simulink model "darko_control_lineaire_lqi"  (R2021b)
settings: Solver=VariableStepAuto  StartTime=0.0  StopTime=30  RelTol=1e-3
values from neighbouring files (symbols this model uses):
  drone = generateDarko()    [main_linearisation.m]
  initial_state = [p_initial; v_initial; q_initial; omega_initial]    [main_linearisation.m]
  K_complet_i = [Ki(:,1:6), zeros(4,1), Ki(:,7:15)]    [main_linearisation.m]
  S_complet_i = [Si(1:6,1:6), zeros(6,1), Si(1:6,7:15); zeros(1,16); Si(7:15,1:6), zeros(9,1), Si(7:15,7:15)]    [main_linearisation.m]
  u_eq = drone.G*drone.MASS/(2*drone.Fb(1,1)) * [1;1;0;0]    [main_linearisation.m]
  x_eq = [[0; 0; 0]; [0; 0; 0]; eul2quat([yaw, pitch, roll])'; [0; 0; 0]]    [main_linearisation.m]
libraries: simulink_extras x11, aerolibanim x1, sharedtransform x1
settings Model: Creator=florian  LastModifiedBy=florian
settings SolverCC: AlgebraicLoopSolver=TrustRegion
settings DebuggingCC: SFMachineParentedDataDiag=warning

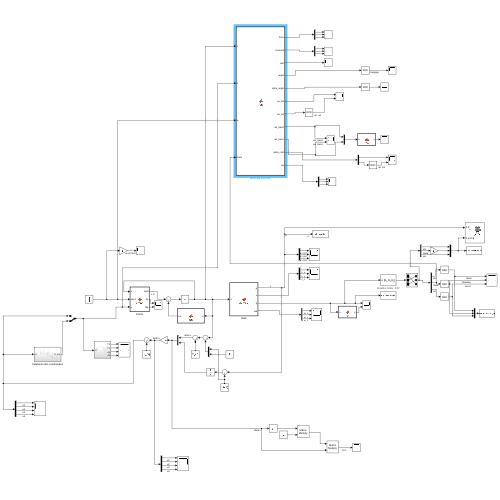
[thumbnail: Simulink's stored preview of the top-level diagram]
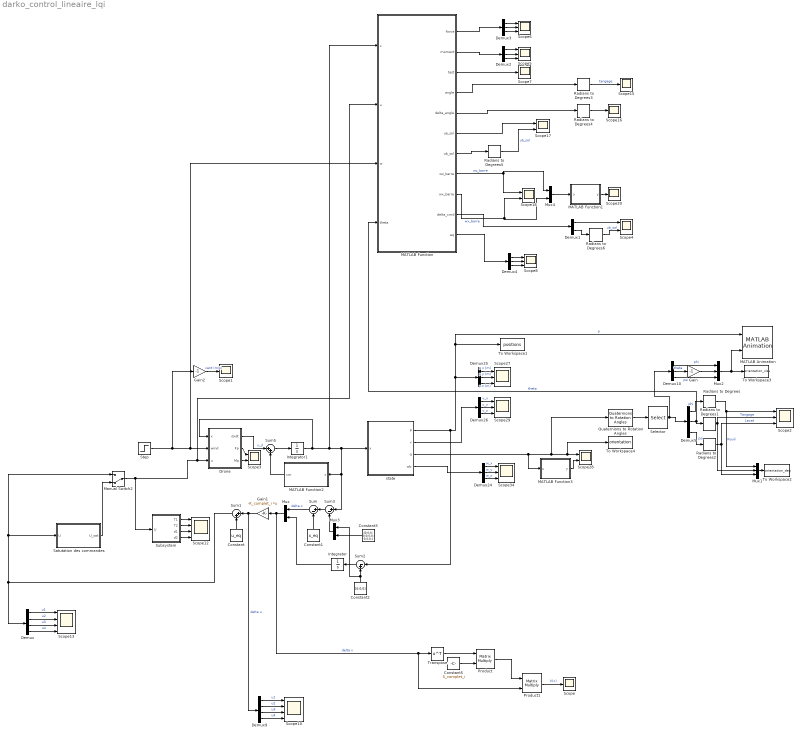
== system darko_control_lineaire_lqi ==
  Constant : Constant  Value=u_eq
  Constant1 : Constant  Value=x_eq
  Constant2 : Constant  Value=[0;0;0]
  Constant3 : Constant  Value=[0;0;0; 0;0;0;0; 0;0;0;]
  Constant5 : Constant  Value=S_complet_i
  Demux : Demux
  Demux1 : Demux  Outputs=2
  Demux{2..5,10,24..26} (8 alike) : Demux  Outputs=3
  Demux9 : Demux
  Drone : MATLAB Function  TreatAsAtomicUnit=on
  Gain : Gain  Gain=-1
  Gain1 : Gain  Gain=-K_complet_i  Multiplication=Matrix(K*u) (u vector)
  Gain2 : Gain  Gain=-1
  Integrator : Integrator  InitialCondition=[0;0;0]
  Integrator1 : Integrator  InitialCondition=initial_state
  MATLAB Animation : aerolibanim/MATLAB Animation  Tag=Matlab Animation 6 DOF  Vehicles=1  Geometries='astredwedge.mat'  BoundingBoxCoordinates=[-50,50,-50,50,-50,50]  CameraOffset=[0,-50,0]  CameraViewAngle=10  SampleTime=0.08  FigurePosition=[635,-23,492,413]
      settings: SourceProductBaseCode=AE
  MATLAB Function : MATLAB Function  TreatAsAtomicUnit=on
  MATLAB Function1 : MATLAB Function  TreatAsAtomicUnit=on
  MATLAB Function2 : MATLAB Function  TreatAsAtomicUnit=on
  MATLAB Function3 : MATLAB Function  TreatAsAtomicUnit=on
  Manual Switch2 : ManualSwitch  CurrentSetting=0
  Mux : Mux  Inputs=2
  Mux1 : Mux  Inputs=3
  Mux2 : Mux  Inputs=3
  Mux3 : Mux  Inputs=2
  Mux4 : Mux  Inputs=2
  Product : Product  Multiplication=Matrix(*)
  Product1 : Product  Multiplication=Matrix(*)
  Quaternions to Rotation Angles : sharedtransform/Quaternions to Rotation Angles  rotationOrder=ZXY  aMode=aMode
      settings: SourceProductBaseCode=AE,PW,DR,MT,UV,VE
  Radians to Degrees{,1..6} (7 alike) : simulink_extras/Transformations/Radians to Degrees
  Satutation des commandes : Subsystem
  Scope{,1,7,15..16,20} (6 alike) : Scope
  Scope10 : Scope  NumInputPorts=4
  Scope12 : Scope  NumInputPorts=4
  Scope13 : Scope  NumInputPorts=4
  Scope{3..4,17..18,28} (5 alike) : Scope  NumInputPorts=2
  Scope{2,5..6,8,27,29,34} (7 alike) : Scope  NumInputPorts=3
  Selector : Selector  InputPortWidth=3  IndexOptions=Index vector (dialog)  Indices=[2 3 1]  OutputSizes=1
  Step : Step  Time=10  Before=[0;0;0]  After=[-1;0;-1]  SampleTime=0
  Subsystem : Subsystem
  Sum : Sum  Inputs=|+-
  Sum1 : Sum  Inputs=|++
  Sum2 : Sum  Inputs=|-+
  Sum3 : Sum  Inputs=|+-
  Sum5 : Sum  Inputs=|++
  To Workspace1 : ToWorkspace  VariableName=positions  SampleTime=-1
  To Workspace2 : ToWorkspace  VariableName=orientation_deg  SampleTime=-1
  To Workspace3 : ToWorkspace  VariableName=orientation_visu  SampleTime=-1
  To Workspace4 : ToWorkspace  VariableName=orientation  SampleTime=-1
  Transpose : Math  Operator=transpose  SaturateOnIntegerOverflow=on
  state : MATLAB Function  TreatAsAtomicUnit=on
  wires:
  Sum5/1 -> Integrator1/1
  MATLAB Function2/1(cor) -> Sum5/2
  Drone/1(dxdt) -> Sum5/1  "x_d"
  Integrator1/1 -> Drone/1(x), MATLAB Function/1(x), state/1(x), Sum3/1, MATLAB Function2/1(x)
  Demux25/3 -> Scope27/3  "p z (m)"
  Demux26/2 -> Scope29/2  "v_y"
  Demux24/1 -> Scope34/1  "w_x"
  MATLAB Function3/1(y) -> Scope28/2
  Demux25/1 -> Scope27/1  "p x (m)"
  state/4(wb) -> Demux24/1
  Demux24/2 -> Scope34/2  "w_y"
  Demux24/3 -> Scope34/3  "w_z"
  state/2(v) -> Demux26/1
  Demux25/2 -> Scope27/2  "p y (m)"
  Demux26/3 -> Scope29/3  "v_z"
  Demux26/1 -> Scope29/1  "v_x"
  Constant/1 -> Sum1/2
  Constant1/1 -> Sum/2
  Demux9/3 -> Scope10/3  "u3"
  Demux9/4 -> Scope10/4  "u4"
  Demux9/1 -> Scope10/1  "u1"
  Demux9/2 -> Scope10/2  "u2"
  Step/1 -> Gain2/1, MATLAB Function/3(w), Drone/2(wind)
  Integrator/1 -> Mux/2
  Sum/1 -> Mux/1  "delta x"
  Demux5/2 -> Radians to Degrees1/1, MATLAB Function/4(theta)  "theta"
  Quaternions to Rotation Angles/1 -> Selector/1
  Demux5/1 -> Radians to Degrees/1  "phi"
  Demux5/3 -> Radians to Degrees2/1  "psi"
  Demux/3 -> Scope13/3  "u3"
  Sum1/1 -> Satutation des commandes/1(U), Manual Switch2/1, Demux/1
  Demux/2 -> Scope13/2  "u2"
  Demux/1 -> Scope13/1  "u1"
  Demux/4 -> Scope13/4  "u4"
  Product1/1 -> Scope/1  "V(x)"
  Gain1/1 -> Demux9/1, Sum1/1  "delta u"
  Product/1 -> Product1/1
  Transpose/1 -> Product/1
  Constant5/1 -> Product/2
  Mux/1 -> Product1/2, Transpose/1, Gain1/1  "delta x"
  Mux1/1 -> To Workspace2/1
  state/3(q) -> Scope28/1, To Workspace4/1, Quaternions to Rotation Angles/1, MATLAB Function3/1(u)
  Satutation des commandes/1(U_sat) -> Manual Switch2/2
  Demux10/2 -> Gain/1  "theta"
  Selector/1 -> Demux10/1, Demux5/1
  Gain/1 -> Mux2/2
  Demux10/1 -> Mux2/1  "phi"
  Demux10/3 -> Mux2/3  "psi"
  state/1(p) -> Sum2/1, Demux25/1, MATLAB Animation/1, To Workspace1/1  "p"
  Mux2/1 -> To Workspace3/1, MATLAB Animation/2
  Gain2/1 -> Scope1/1  "vent (m/s)"
  Radians to Degrees1/1 -> Scope2/2, Mux1/2  "Tangage"
  Radians to Degrees/1 -> Scope2/1, Mux1/1  "Rouli"
  Radians to Degrees2/1 -> Scope2/3, Mux1/3  "Lacet"
  Sum2/1 -> Integrator/1
  Constant2/1 -> Mux3/1, Sum2/2
  Sum3/1 -> Sum/1
  Mux3/1 -> Sum3/2
  Constant3/1 -> Mux3/2
  Drone/2(Fp) -> Scope3/1
  Drone/3(Mp) -> Scope3/2
  Manual Switch2/1 -> Subsystem/1(U), MATLAB Function/2(u), Drone/3(u)
  Subsystem/3(d1) -> Scope12/3
  Subsystem/4(d2) -> Scope12/4
  Subsystem/2(T2) -> Scope12/2
  Subsystem/1(T1) -> Scope12/1
  Mux4/1 -> MATLAB Function1/1(u)
  MATLAB Function/7(ub_sol) -> Radians to Degrees5/1
  MATLAB Function/5(delta_angle) -> Radians to Degrees4/1
  Radians to Degrees3/1 -> Scope15/1  "tangage"
  MATLAB Function1/1(y) -> Scope20/1
  MATLAB Function/4(angle) -> Radians to Degrees3/1
  Radians to Degrees4/1 -> Scope16/1
  Radians to Degrees5/1 -> Scope17/2  "ub_sol"
  MATLAB Function/9(wx_barre) -> Scope18/2, Mux4/2  "wx_barre"
  MATLAB Function/8(wz_barre) -> Scope18/1, Mux4/1  "wz_barre"
  MATLAB Function/6(ua_sol) -> Scope17/1
  MATLAB Function/10(delta_cmd) -> Demux1/1
  Demux1/1 -> Scope4/1
  Demux2/1 -> Scope5/1
  Demux2/2 -> Scope5/2
  Demux2/3 -> Scope5/3
  MATLAB Function/2(moment) -> Demux2/1
  Demux3/1 -> Scope6/1
  Demux3/2 -> Scope6/2
  Demux3/3 -> Scope6/3
  MATLAB Function/1(force) -> Demux3/1
  MATLAB Function/3(test) -> Scope7/1
  Radians to Degrees6/1 -> Scope4/2  "ub_sol"
  Demux1/2 -> Radians to Degrees6/1
  Demux4/1 -> Scope8/1
  Demux4/2 -> Scope8/2
  Demux4/3 -> Scope8/3
  MATLAB Function/11(eq) -> Demux4/1

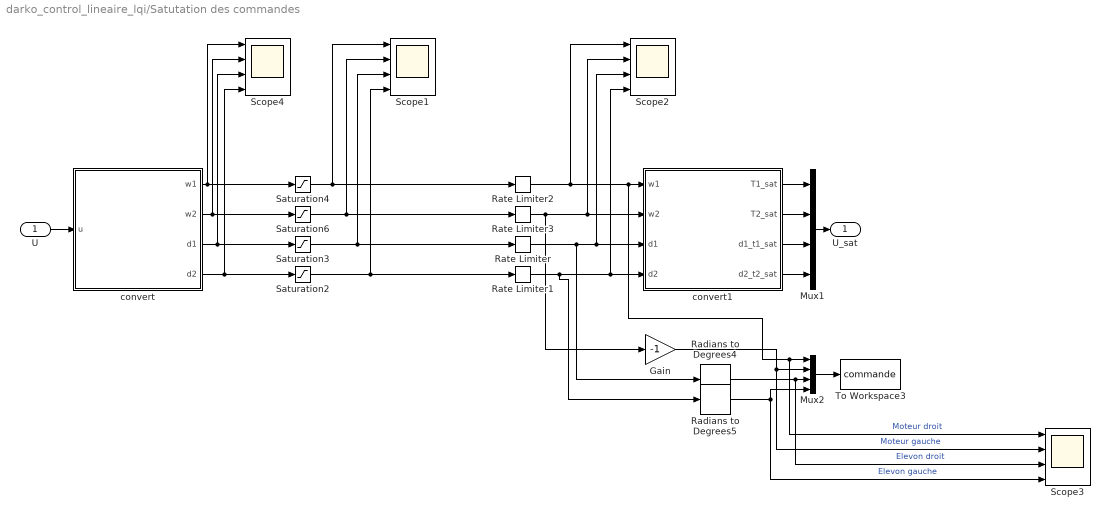
== system darko_control_lineaire_lqi/Satutation des commandes ==
  U : Inport
  Gain : Gain  Gain=-1
  Mux1 : Mux
  Mux2 : Mux
  Radians to Degrees4 : simulink_extras/Transformations/Radians to Degrees
  Radians to Degrees5 : simulink_extras/Transformations/Radians to Degrees
  Rate Limiter : RateLimiter  RisingSlewLimit=drone.ELEVON_RATE_CHANGE  FallingSlewLimit=-drone.ELEVON_RATE_CHANGE  SampleTimeMode=inherited
  Rate Limiter1 : RateLimiter  RisingSlewLimit=drone.ELEVON_RATE_CHANGE  FallingSlewLimit=-drone.ELEVON_RATE_CHANGE  SampleTimeMode=inherited
  Rate Limiter2 : RateLimiter  RisingSlewLimit=drone.MOTOR_RATE_CHANGE  FallingSlewLimit=-drone.MOTOR_RATE_CHANGE  SampleTimeMode=inherited
  Rate Limiter3 : RateLimiter  RisingSlewLimit=drone.MOTOR_RATE_CHANGE  FallingSlewLimit=-drone.MOTOR_RATE_CHANGE  SampleTimeMode=inherited
  Saturation2 : Saturate  UpperLimit=30*(pi/180)  LowerLimit=-30*(pi/180)
  Saturation3 : Saturate  UpperLimit=30*(pi/180)  LowerLimit=-30*(pi/180)
  Saturation4 : Saturate  UpperLimit=1000  LowerLimit=200
  Saturation6 : Saturate  UpperLimit=1000  LowerLimit=200
  Scope{1..4} (4 alike) : Scope  NumInputPorts=4
  To Workspace3 : ToWorkspace  VariableName=commande  SampleTime=-1
  convert : MATLAB Function  TreatAsAtomicUnit=on
  convert1 : MATLAB Function  TreatAsAtomicUnit=on
  U_sat : Outport
  wires:
  convert/1(w1) -> Saturation4/1, Scope4/1
  Saturation3/1 -> Rate Limiter/1, Scope1/3
  convert/2(w2) -> Scope4/2, Saturation6/1
  convert/3(d1) -> Scope4/3, Saturation3/1
  convert/4(d2) -> Saturation2/1, Scope4/4
  convert1/1(T1_sat) -> Mux1/1
  convert1/4(d2_t2_sat) -> Mux1/4
  Mux1/1 -> U_sat/1
  convert1/2(T2_sat) -> Mux1/2
  convert1/3(d1_t1_sat) -> Mux1/3
  Saturation2/1 -> Rate Limiter1/1, Scope1/4
  Saturation6/1 -> Rate Limiter3/1, Scope1/2
  Saturation4/1 -> Rate Limiter2/1, Scope1/1
  U/1 -> convert/1(u)
  Radians to Degrees5/1 -> Mux2/4, Scope3/4  "Elevon gauche"
  Rate Limiter3/1 -> Gain/1, convert1/2(w2), Scope2/2
  Rate Limiter1/1 -> Radians to Degrees5/1, Scope2/4, convert1/4(d2)
  Rate Limiter/1 -> Radians to Degrees4/1, Scope2/3, convert1/3(d1)
  Gain/1 -> Scope3/2, Mux2/2  "Moteur gauche"
  Mux2/1 -> To Workspace3/1
  Radians to Degrees4/1 -> Scope3/3, Mux2/3  "Elevon droit"
  Rate Limiter2/1 -> Scope2/1, Scope3/1, Mux2/1, convert1/1(w1)  "Moteur droit"

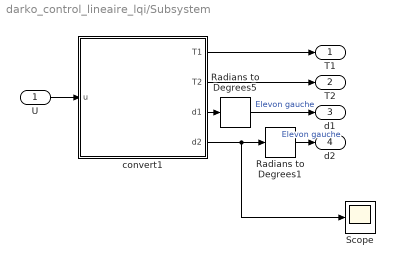
== system darko_control_lineaire_lqi/Subsystem ==
  U : Inport
  Radians to Degrees1 : simulink_extras/Transformations/Radians to Degrees
  Radians to Degrees5 : simulink_extras/Transformations/Radians to Degrees
  Scope : Scope
  convert1 : MATLAB Function  TreatAsAtomicUnit=on
  T1 : Outport
  T2 : Outport  Port=2
  d1 : Outport  Port=3
  d2 : Outport  Port=4
  wires:
  U/1 -> convert1/1(u)
  convert1/1(T1) -> T1/1
  convert1/2(T2) -> T2/1
  Radians to Degrees5/1 -> d1/1  "Elevon gauche"
  convert1/3(d1) -> Radians to Degrees5/1
  Radians to Degrees1/1 -> d2/1  "Elevon gauche"
  convert1/4(d2) -> Scope/1, Radians to Degrees1/1

== matlab function darko_control_lineaire_lqi/MATLAB Function2 ==
  data: x input; cor output
function cor  = fcn(x)
%#codegen
q  = x(7:10);
n = norm(q);
mismatch = 1-n;
cor = [0;0;0; 0;0;0; mismatch*q; 0;0;0];

== matlab function darko_control_lineaire_lqi/MATLAB Function3 ==
  data: u input; y output
function y = fcn(u)
%#codegen

y = norm(u);

== matlab function darko_control_lineaire_lqi/state ==
  data: x input; p output; v output; q output; wb output
function [p, v, q, wb] = demux(x)
%#codegen

p = x(1:3);
v = x(4:6);
q  = x(7:10);
wb = x(11:13);

== matlab function darko_control_lineaire_lqi/MATLAB Function ==
  data: force output; moment output; test output; x input; u input; w input; theta input; drone parameter; angle output; delta_angle output; ua_sol output; ub_sol output; wz_barre output; wx_barre output; delta_cmd output; eq output
function [force,moment, test, angle, delta_angle, ua_sol, ub_sol, wz_barre, wx_barre, delta_cmd, eq] = fcn(x, u, w, theta, drone)
%#codegen


% p = x(1:3);
vl = x(4:6);
q  = x(7:10);
wb = x(11:13);

PHI_fv = drone.PHI(1:3,1:3);
PHI_mv = drone.PHI(4:6,1:3);
PHI_mw = drone.PHI(4:6,4:6);
phi_n  = drone.PHI_n;
rho    = drone.RHO;
Swet   = drone.WET_SURFACE;
Sdry   = drone.DRY_SURFACE;
chord  = drone.CHORD;
ws     = drone.WINGSPAN;
xi_m = drone.ELEVON_MEFFICIENCY;
xi_f = drone.ELEVON_FEFFICIENCY;
a1 = drone.P_A1_CG;
a2 = drone.P_A2_CG;
Sp = pi*drone.PROP_RADIUS^2;
dR = drone.CENTRAGE ;

% gravity
g = drone.G;
% vehicle mass
m = drone.MASS;

cd0 = PHI_fv(1,1);
cl0 = PHI_fv(3,3);

S = Swet + Sdry;

D = q2dcm(q);

B = diag([ws; chord; ws]);
vinf = D'*(vl-w);

eta = sqrt( norm(vinf)^2 + phi_n*norm(B*wb)^2 );


T1 = max(u(1),0);
T2 = max(u(2),0);
d1_T1 = u(3);
d2_T2 = u(4);

d1 = d1_T1/T1;
d2 = d2_T2/T2;

ua = T1;
ub = d1;

eq1 = 2*(1-(S/(4*Sp))*cd0)*ua - 1/2*rho*S*eta*cd0*vinf(1) + 1/2*rho*S*eta*cd0*xi_f(2)*ub*vinf(3) - m*g*sin(theta);

eq2 = -1/2*rho*S*eta*cl0*vinf(3) - 1/2*rho*S*eta*cl0*xi_f(2)*ub*vinf(1) - S/(2*Sp)*xi_f(2)*cl0*ua*ub + m*g*cos(theta);

eq3 = 1/2*rho*S*dR*cl0*eta*vinf(3) + 1/2*rho*S*dR*cl0*eta*xi_m(2)*ub*vinf(1) + S/(2*Sp)*dR*cl0*xi_m(2)*ua*ub;


Fp = -1/2 * rho * S * PHI_fv * eta * vinf ...
     + 1/4 * rho * S * PHI_fv * skew_sym(xi_f) * (d1 + d2) * eta * vinf + drone.Fb*u +D'*[0;0;m*g]-1/2 * rho * S * PHI_mv * eta * B * wb + 1/4 * rho * S * PHI_mv * skew_sym(xi_f) * (d1 + d2) * B * eta * wb;

Mp = -1/2 * rho * S * B * PHI_mv * eta * vinf  ...
     + 1/4 * rho * S * skew_sym(a1) * PHI_fv * skew_sym(xi_f)* d1 * eta * vinf ...
     + 1/4 * rho * S * skew_sym(a2) * PHI_fv * skew_sym(xi_f)* d2 * eta * vinf ...
     + 1/4 * rho * S * B * PHI_mv * skew_sym(xi_m) * (d1 + d2) * eta * vinf ...
      +drone.Mb*u + 1/4 * rho * S * B * PHI_mw * skew_sym(xi_m) * (d1 + d2) * eta * B * wb - 1/2 * rho * S *B * PHI_mw * eta * wb + 1/4 * rho * S * skew_sym(a1) * PHI_mv * skew_sym(xi_f)* d1 * eta * B * eta * wb + 1/4 * rho * S * skew_sym(a2) * PHI_mv * skew_sym(xi_f)* d2 * eta * B * eta * wb; 

temp = drone.Fb*u;
test =  2*(1-(S/(4*Sp))*cd0)*ua - temp(1);


force = [eq1;0;eq2] - Fp;
moment = [0;eq3;0] - Mp;


eta2 = norm(w);


if eta2 ~= 0
    
%     angle =  [2*atan((b_theta-sqrt(a_theta^2 + b_theta^2))/a_theta), 2*atan((b_theta+sqrt(a_theta^2 + b_theta^2))/a_theta)]; % 
    angle = -atan(w(3)/w(1) - (2*m*g)/(rho*S*cl0*eta2*((xi_f(2)/xi_m(2))-1)*w(1)));

    
    delta_angle = theta -  angle;

    w_barre  = [cos(angle), 0, -sin(angle); 0, 1, 0; sin(angle), 0, cos(angle)]*(-w);
    wx_barre = w_barre(1);
    wz_barre = w_barre(3);


    a = 2*(1-(S*cd0)/(4*Sp));
    b = 1/2*rho*S*eta2*cd0*xi_f(2)*wz_barre;
    c = -1/2*rho*S*eta2*cd0*wx_barre - m*g*sin(angle);

    d =  -1/2*rho*S*eta2*cl0*xi_f(2)*wx_barre;
    e = - S/(2*Sp)*xi_f(2)*cl0;
    f = -1/2*rho*S*eta2*cl0*wz_barre + m*g*cos(angle);
% 
%     ua_sol = (-sqrt(a^2*d^2 + 4*e*a*b*f + 2*e*a*c*d + e^2*c^2) - a*d + e*c)/(2*e*a);
%     ub_sol = (sqrt(a^2*d^2 + 4*e*a*b*f + 2*e*a*c*d + e^2*c^2) + a*d + e*c)/(2*e*b);
    ua_sol = -(sqrt(a^2*d^2 + 4*e*a*b*f + 2*e*a*c*d + e^2*c^2) - a*d + e*c)/(2*e*a);
    ub_sol = -(-sqrt(a^2*d^2 + 4*e*a*b*f + 2*e*a*c*d + e^2*c^2) + a*d + e*c)/(2*e*b);
    delta_cmd = [ua;ub]- [ua_sol;ub_sol];


    eq = [2*(1-(S/(4*Sp))*cd0)*ua_sol - 1/2*rho*S*eta*cd0*vinf(1) + 1/2*rho*S*eta*cd0*xi_f(2)*ub_sol*vinf(3) - m*g*sin(angle);...
          -1/2*rho*S*eta*cl0*vinf(3) - 1/2*rho*S*eta*cl0*xi_f(2)*ub_sol*vinf(1) - S/(2*Sp)*xi_f(2)*cl0*ua_sol*ub_sol + m*g*cos(angle);...
          1/2*rho*S*dR*cl0*eta*vinf(3) + 1/2*rho*S*dR*cl0*eta*xi_m(2)*ub_sol*vinf(1) + S/(2*Sp)*dR*cl0*xi_m(2)*ua_sol*ub_sol ];

else
    wx_barre = 0;
    wz_barre = 0;
    angle = 0;
    delta_angle = 0;
    ua_sol = 0;
    ub_sol = 0;
    delta_cmd = [0;0];
    eq = [0;0;0];
end

== matlab function darko_control_lineaire_lqi/Drone ==
  data: x input; wind input; u input; dxdt output; drone parameter; Fp output; Mp output
function [dxdt,Fp,Mp] = drone(x,wind, u, drone)

%% physical constants
% gravity
g = drone.G;
% vehicle mass
m = drone.MASS;
% vehicle inertia matrix
J = drone.INERTIA; % [3x3 real symmetric] in body axis

%% state demultiplexing
% p = x(1:3);
v = x(4:6);
q  = x(7:10);
wb = x(11:13);

Rq = q2dcm(q);

[Fp, Mp] = external_force_moment(x, u, wind, drone);

% position
dpdt = v;

% kinematics
dvdt =  [0;0;g] + (1/m)*Rq*drone.Fb*u + (1/m)*Rq*Fp; 

%% quaternion derivative
eta = q(1);
eps = q(2:4);

dqdt = (1/2)*[-eps'; eta*eye(3) + skew_sym(eps)]*wb;

%% angular velocity derivative
% kinematics
dwdt = -J\cross(wb, J*wb) + J\(drone.Mb*u) + J\Mp;


%% derivative multiplexing
dxdt = [dpdt; dvdt; dqdt; dwdt] ;

== matlab function darko_control_lineaire_lqi/Subsystem/convert1 ==
  data: u input; T1 output; drone parameter; T2 output; d1 output; d2 output
function [T1, T2, d1, d2] = convert(u, drone)
%#codegen
kf = drone.PROP_KP;

T1 = max(u(1),0);
T2 = max(u(2),0);
d1_T1 = u(3);
d2_T2 = u(4);

w1 = sqrt(T1/kf);
w2 = sqrt(T2/kf);
d1 = d1_T1/T1;
d2 = d2_T2/T2;

== matlab function darko_control_lineaire_lqi/MATLAB Function1 ==
  data: u input; y output
function y = fcn(u)
%#codegen

y = norm(u);

== matlab function darko_control_lineaire_lqi/Satutation des commandes/convert ==
  data: u input; w1 output; drone parameter; w2 output; d1 output; d2 output
function [w1, w2, d1, d2] = convert(u, drone)
%#codegen
kf = drone.PROP_KP;

T1 = max(u(1),0);
T2 = max(u(2),0);
d1_T1 = u(3);
d2_T2 = u(4);

w1 = sqrt(T1/kf);
w2 = sqrt(T2/kf);
d1 = d1_T1/T1;
d2 = d2_T2/T2;

== matlab function darko_control_lineaire_lqi/Satutation des commandes/convert1 ==
  data: w1 input; w2 input; d1 input; d2 input; T1_sat output; T2_sat output; drone parameter; d1_t1_sat output; d2_t2_sat output
function [T1_sat, T2_sat, d1_t1_sat, d2_t2_sat] = convert2(w1, w2, d1, d2, drone)
%#codegen
kf = drone.PROP_KP;

T1_sat = kf*w1^2;
d1_t1_sat = d1*T1_sat;
T2_sat = kf*w2^2;
d2_t2_sat = d2*T2_sat;
